simulink model "case_7_lead_slow_down_then_steady"  (R2025a)
settings: Solver=VariableStepAuto  StartTime=0.0  StopTime=10  RelTol=1e-3
settings Model: Creator=sanborkl  LastModifiedBy=admin

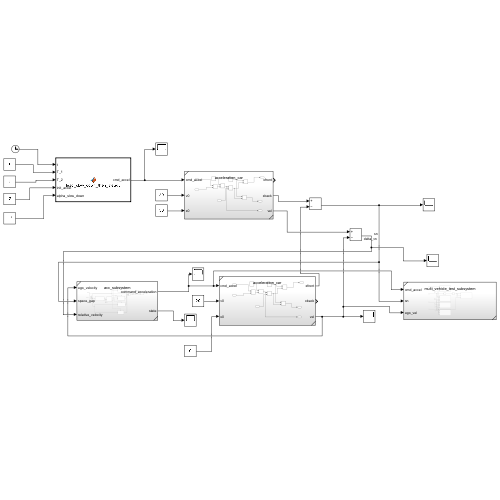
[thumbnail: Simulink's stored preview of the top-level diagram]
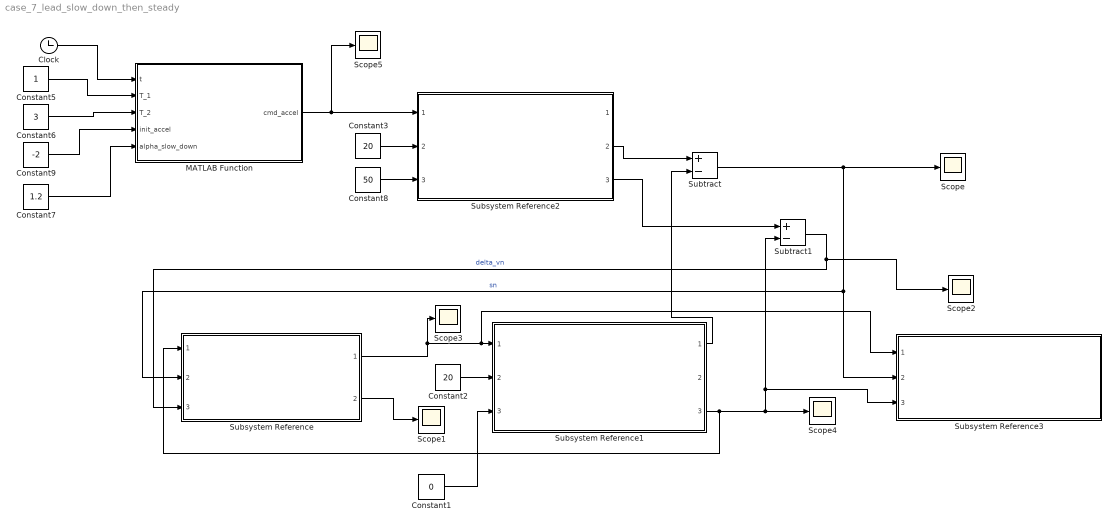
== system case_7_lead_slow_down_then_steady ==
  Clock : Clock
  Constant1 : Constant  Value=0
  Constant2 : Constant  Value=20
  Constant3 : Constant  Value=20
  Constant5 : Constant
  Constant6 : Constant  Value=3
  Constant7 : Constant  Value=1.2
  Constant8 : Constant  Value=50
  Constant9 : Constant  Value=-2
  MATLAB Function : MATLAB Function  TreatAsAtomicUnit=on
  Scope{,1..5} (6 alike) : Scope
      Scope settings: ActiveDisplayYMinimum=34.013496751198524  ActiveDisplayYMaximum=46.857499375639875
      Scope1 settings: ActiveDisplayYMinimum=-1  ActiveDisplayYMaximum=1  DataLoggingVariableName=ScopeData2
      Scope2 settings: ActiveDisplayYMinimum=-4.7594091268070251  ActiveDisplayYMaximum=1.3400896063993253  DataLoggingVariableName=ScopeData3
      Scope3 settings: ActiveDisplayYMinimum=-2.2847275709033061  ActiveDisplayYMaximum=2.4791026840062962  DataLoggingVariableName=ScopeData4
      Scope4 settings: ActiveDisplayYMinimum=-1  ActiveDisplayYMaximum=1
      Scope5 settings: ActiveDisplayYMinimum=-4.7098976656641858  ActiveDisplayYMaximum=2.943215908942431  DataLoggingVariableName=ScopeData5
  Subsystem Reference : Subsystem  ReferencedSubsystem=acc_subsystem
  Subsystem Reference1 : Subsystem  ReferencedSubsystem=acceleration_car
  Subsystem Reference2 : Subsystem  ReferencedSubsystem=acceleration_car
  Subsystem Reference3 : Subsystem  ReferencedSubsystem=multi_vehicle_test_subsystem
  Subtract : Sum  Inputs=+-
  Subtract1 : Sum  Inputs=+-
  wires:
  Subsystem Reference2/3 -> Subtract1/1
  Constant3/1 -> Subsystem Reference2/2
  Constant2/1 -> Subsystem Reference1/2
  Subsystem Reference1/1 -> Subtract/2
  Subsystem Reference/1 -> Scope3/1, Subsystem Reference3/1, Subsystem Reference1/1
  Constant1/1 -> Subsystem Reference1/3
  Subsystem Reference/2 -> Scope1/1
  Subsystem Reference2/2 -> Subtract/1
  Subtract/1 -> Subsystem Reference3/2, Subsystem Reference/2, Scope/1  "sn"
  Subsystem Reference1/3 -> Subsystem Reference/1, Subtract1/2, Subsystem Reference3/3, Scope4/1
  Subtract1/1 -> Scope2/1, Subsystem Reference/3  "delta_vn"
  Clock/1 -> MATLAB Function/1(t)
  Constant5/1 -> MATLAB Function/2(T_1)
  Constant6/1 -> MATLAB Function/3(T_2)
  Constant7/1 -> MATLAB Function/5(alpha_slow_down)
  Constant8/1 -> Subsystem Reference2/3
  Constant9/1 -> MATLAB Function/4(init_accel)
  MATLAB Function/1(cmd_accel) -> Scope5/1, Subsystem Reference2/1

== matlab function case_7_lead_slow_down_then_steady/MATLAB Function ==
  data: t input; cmd_accel output; T_1 input; T_2 input; init_accel input; alpha_slow_down input
function cmd_accel = lead_slow_down_then_steady(t, T_1, T_2, init_accel , alpha_slow_down)
% alpha_slow_down is how fast the lead car is slowing down, 

if t < T_1
    cmd_accel = init_accel;
elseif (T_1 <= t) && (t < T_2)
    cmd_accel = max(init_accel + -(alpha_slow_down * t), 0);
else
    cmd_accel = 0;
end
